simulink model "Copy_of_newCommunication"  (R2025a)
settings: Solver=VariableStepAuto  StartTime=0.0  StopTime=Inf  RelTol=1e-3
values from neighbouring files (symbols this model uses):
  Boom_Cmd_LUT = joints(1).lut_y    [LUT.m]
  Boom_Vel_LUT = joints(1).lut_x    [LUT.m]
  Stick_Cmd_LUT = joints(2).lut_y    [LUT.m]
  Stick_Vel_LUT = joints(2).lut_x    [LUT.m]
undefined symbols (not defined in the file or in its folder): canChannel
libraries: canlib x10, canmsglib x8, simulink x8, eeGeneralControl x5, simulink_extras x4, slpidlib x2, sl3dlib x1
settings Model: Creator=Viktor Traktor  LastModifiedBy=Viktor Traktor

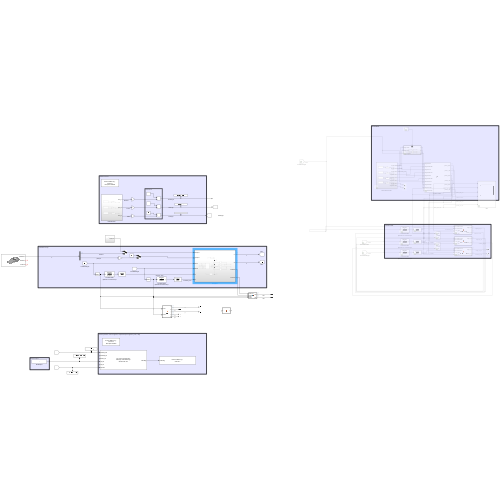
[thumbnail: Simulink's stored preview of the top-level diagram]
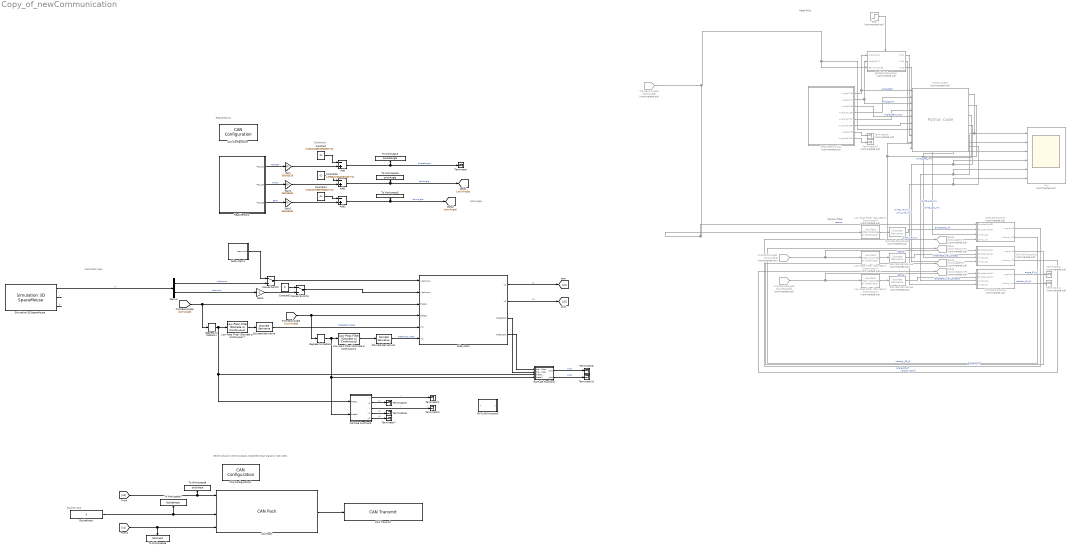
== system Copy_of_newCommunication ==
  note: Controller Loop
  note: bomAngle
  note: Calibration
  note: Send hydraulic control signals, expected input signals [-100, 100]
  note: Read sensors
  note: Bucket Input
  note: Kalman Filter
  note: Read IMUs
  Add : Sum  Inputs=-+
  Add1 : Sum  Inputs=-+
  Add2 : Sum  Inputs=-+
  BucketInput : Constant  Value=0
  CAN Configuration : canlib/CAN Configuration  BlockHandle=17154.0007  Device=Kvaser USBcan Light 1 (Channel 1)  DeviceMenu=Kvaser USBcan Light 1 (Channel 1)  ObjConstructor=canChannel('Kvaser', 'USBcan Light 1', 1)  BusSpeed=500000  EnableBitParameters=off  SJW=1  TSEG1=4  TSEG2=3  NSamples=1  AckMode=Normal
  CAN Configuration1 : canlib/CAN Configuration  BlockHandle=17155.0007  Device=Kvaser USBcan Light 1 (Channel 2)  DeviceMenu=Kvaser USBcan Light 1 (Channel 2)  ObjConstructor=canChannel('Kvaser', 'USBcan Light 1', 2)  BusSpeed=500000  EnableBitParameters=off  SJW=1  TSEG1=4  TSEG2=3  NSamples=1  AckMode=Normal
  CAN Pack : canmsglib/CAN Pack  CANdbFile=C:\Users\Viktor Traktor\IQAN\ec20_hydraulics.dbc  MsgList=ControlMessage  MsgName=ControlMessage  MsgIDType=Standard (11-bit identifier)  MsgIdentifier=387  CANIDInput=off  MsgLength=6  Remote=off  ApplyMinMax=off  BusOutput=off  SignalInfo={'Parallell_FR','8','8','LE','signed','Standard','0','1','0','-Inf','Inf';'Parallelll_RL','0','8','LE','signed','Standard','0','1','0','-Inf','Inf';'Rotate_RL','40','8','LE','signed','Standard','0','1','0','-Inf','Inf';'Tilt_FR','24','8','LE','signed','Standard','0','1','0','-Inf','Inf';'Tilt_RL','32','8','LE','signed','Standard','0','1','0','-Inf','Inf';'UpDown','16','8','LE','signed','Standard','0','1','0','-Inf','Inf'}
      settings: LibrarySourceBlock=canlib/CAN Pack  DataFormat=CANdb specified signals
  CAN Transmit : canlib/CAN Transmit  BlockHandle=17164.0007  Device=Kvaser USBcan Light 1 (Channel 2)  DeviceMenu=Kvaser USBcan Light 1 (Channel 2)  ObjConstructor=canChannel('Kvaser', 'USBcan Light 1', 2)  EnableEventTransmit=off  EnablePeriodicTransmit=off  MessagePeriod=1.000
  Constant : Constant  Value=2.060410383456638e+02
  Constant1 : Constant  Value=2.052407368979854e+02
  Constant2 : Constant  Value=0
  Constant5 : Constant  Value=2.390501084826040e+02
  Degrees to Radians : simulink_extras/Transformations/Degrees to Radians
  Degrees to Radians1 : simulink_extras/Transformations/Degrees to Radians
  Demux : Demux  Outputs=2
  Discrete Derivative : simulink/Discrete/Discrete Derivative  gainval=1.0  ICPrevScaledInput=0.0  OutMin=[]  OutMax=[]  OutDataType=fixdt(1, 16)  OutScaling=2^-10  DoSatur=off
  Discrete Derivative1 : simulink/Discrete/Discrete Derivative  gainval=1.0  ICPrevScaledInput=0.0  OutMin=[]  OutMax=[]  OutDataType=fixdt(1, 16)  OutScaling=2^-10  DoSatur=off
  Discrete Derivative2 : simulink/Discrete/Discrete Derivative  Commented=on  gainval=1.0  ICPrevScaledInput=0.0  OutMin=[]  OutMax=[]  OutDataType=fixdt(1, 16)  OutScaling=2^-10  DoSatur=off
  Discrete Derivative3 : simulink/Discrete/Discrete Derivative  Commented=on  gainval=1.0  ICPrevScaledInput=0.0  OutMin=[]  OutMax=[]  OutDataType=fixdt(1, 16)  OutScaling=2^-10  DoSatur=off
  Discrete Derivative4 : simulink/Discrete/Discrete Derivative  Commented=on  gainval=1.0  ICPrevScaledInput=0.0  OutMin=[]  OutMax=[]  OutDataType=fixdt(1, 16)  OutScaling=2^-10  DoSatur=off
  Enabled Subsystem : Subsystem  Commented=on  TreatAsAtomicUnit=on
  FromBomAngle1 : From  Commented=on  GotoTag=bomAngle
  FromBucketAngle : From  Commented=on  GotoTag=bucketAngle
  FromStickAngle1 : From  Commented=on  GotoTag=stickAngle
  Gain : Gain  Gain=360/65535
  Gain1 : Gain  Gain=360/65535
  Gain2 : Gain  Gain=360/65535
  Gain3 : Gain  Gain=-1
  Goto3 : Goto  Commented=on  GotoTag=bomAngleKF
  Goto4 : Goto  Commented=on  GotoTag=bomVelocityKF
  Goto5 : Goto  Commented=on  GotoTag=stickAngleKF
  Goto6 : Goto  Commented=on  GotoTag=stickVelocityKF
  IMU : Scope  Commented=on  NumInputPorts=6
      settings: ActiveDisplayYMinimum=240.03476604985391  ActiveDisplayYMaximum=241.62685406904103
  Low-Pass Filter (Discrete or Continuous)1 : eeGeneralControl/Low-Pass Filter (Discrete or Continuous)  K=1  T=.15  B=inf  A=-inf  init_option=Inherited from block input  x0=0  Ts=0.1
  Low-Pass Filter (Discrete or Continuous)4 : eeGeneralControl/Low-Pass Filter (Discrete or Continuous)  Commented=on  K=1  T=.15  B=inf  A=-inf  init_option=Inherited from block input  x0=0  Ts=0.1
  Low-Pass Filter (Discrete or Continuous)5 : eeGeneralControl/Low-Pass Filter (Discrete or Continuous)  Commented=on  K=1  T=.15  B=inf  A=-inf  init_option=Inherited from block input  x0=0  Ts=0.1
  Low-Pass Filter (Discrete or Continuous)6 : eeGeneralControl/Low-Pass Filter (Discrete or Continuous)  Commented=on  K=1  T=.15  B=inf  A=-inf  init_option=Inherited from block input  x0=0  Ts=0.1
  Low-Pass Filter (Discrete or Continuous)7 : eeGeneralControl/Low-Pass Filter (Discrete or Continuous)  K=1  T=.15  B=inf  A=-inf  init_option=Inherited from block input  x0=0  Ts=0.1
  MATLAB Function : MATLAB Function  Commented=on  TreatAsAtomicUnit=on
  MATLAB Function1 : MATLAB Function  Commented=on  TreatAsAtomicUnit=on
  MATLAB Function2 : MATLAB Function  Commented=on  TreatAsAtomicUnit=on
  MATLAB Function3 : MATLAB Function  TreatAsAtomicUnit=on
  MATLAB Function4 : MATLAB Function  TreatAsAtomicUnit=on
  MATLAB Function5 : MATLAB Function  TreatAsAtomicUnit=on
  Manual Switch : ManualSwitch
  Manual Switch1 : ManualSwitch
  Python Code1 : PythonCode  Commented=on  OutputCode=|  SampleTime=0.01
      | # Computation
      | 
      | #print(Angle128X)
      | 
      | if Angle128X > 180:
      |     Angle128X = abs(Angle128X) - 360
      |     
      | if Angle137X < 20:
      |     Angle137X = abs(Angle137X)+360
      |     
      | if Angle138X > 270:
      |     Angle138X = abs(Angle138X) - 360
      |     
      | #print("///")
      | #print(Angle128X)
      | 
      | print(Angle128Xp)
      | print(Angle137Xp)
      | print(Encoder33Xp)
      |     
      | joint1_pos = Angle137X -270 + Angle128X - (Angle137Xp-270 + Angle128Xp - Encoder33Xp)
      | joint1_vel = -(AngleVel137X - AngleVel128X)
      | 
      | joint2_pos = 180 + (90 - joint1_pos) + Angle138X
      | joint2_vel = AngleVel138X - joint1_vel
      | 
      | joint3_pos = 0
      | joint3_vel = 0
  Read Sensors : Subsystem
  Read Sensors IMU : Subsystem  Commented=on
  Simulation 3D SpaceMouse : sl3dlib/Simulation 3D/Hardware Interface/Simulation 3D SpaceMouse  Port=USB1  OutputType=Speed  Dominant=off  DisableTranslation=off  DisableRotation=off  NormalizeAngle=off  EnableLimit=off  PositionSensitivity=0.00058  RotationSensitivity=0.00001  InitialPosition=[0 0 0]  InitialRotation=[0 0 1 0]  PositionLow=[-100 -100 -100]  PositionUp=[100 100 100]
  Step : Step  Commented=on  Time=0.001  Before=1  After=0  SampleTime=0
  Subsystem : Subsystem
  Subsystem1 : Subsystem
  Terminator{,1,3,5..8,11} (8 alike) : Terminator
  Terminator{2,4,9..10} (4 alike) : Terminator  Commented=on
  To Workspace : ToWorkspace  VariableName=bucketAngle  SaveFormat=Timeseries  SampleTime=-1
  To Workspace1 : ToWorkspace  VariableName=stickAngle  SaveFormat=Timeseries  SampleTime=-1
  To Workspace2 : ToWorkspace  VariableName=bomAngle  SaveFormat=Timeseries  SampleTime=-1
  To Workspace6 : ToWorkspace  VariableName=bomInput  SaveFormat=Timeseries  SampleTime=-1
  To Workspace7 : ToWorkspace  VariableName=bucketInput  SaveFormat=Timeseries  SampleTime=-1
  To Workspace8 : ToWorkspace  VariableName=stickInput  SaveFormat=Timeseries  SampleTime=-1
  wires:
  BucketInput/1 -> CAN Pack/4, To Workspace7/1
  Add2/1 -> [bomAngle], To Workspace2/1  "bomAngle"
  Constant1/1 -> Add2/1
  Gain/1 -> Add/2
  Read Sensors/2(Pos_20) -> Gain1/1  "STICK"
  [u2] -> CAN Pack/1, To Workspace8/1
  Constant/1 -> Add/1
  Read Sensors/1(Pos_01) -> Gain/1  "BUCKET"
  Gain2/1 -> Add2/2
  Read Sensors/3(Pos_33) -> Gain2/1  "BOM"
  CAN Pack/1 -> CAN Transmit/1
  Add/1 -> Terminator/1, To Workspace/1  "bucketAngle"
  [u1] -> CAN Pack/6, To Workspace6/1
  Add1/1 -> [stickAngle], To Workspace1/1  "stickAngle"
  MATLAB Function1/2(velocity_20) -> Goto6/1  "velocity_20_kf"
  Enabled Subsystem/1(Out1) -> Python Code1/8
  Discrete Derivative2/1 -> MATLAB Function/2(EncoderVel33X)  "Encoder33_vel"
  MATLAB Function/1(angle_33) -> Goto3/1  "angle_33_kf"
  Read Sensors IMU/3(Angle138X) -> Python Code1/5  "Angle138X_input"
  Python Code1/4 -> MATLAB Function1/4(joint2_vel), IMU/4  "join2_vel_imu"
  Read Sensors IMU/4(AngleVel128X) -> Python Code1/2
  Read Sensors IMU/1(Angle128X) -> Python Code1/1, Enabled Subsystem/1(Angle128X)  "Angle128X"
  Read Sensors IMU/8(AngleVel139X) -> Terminator10/1
  Python Code1/3 -> IMU/3, MATLAB Function1/3(joint2_pos)  "joint2_pos_imu"
  Python Code1/5 -> MATLAB Function2/3(joint3_pos), IMU/5  "joint3_pos_imu"
  MATLAB Function/2(velocity_33) -> Goto4/1  "velocity_33_kf"
  Python Code1/6 -> MATLAB Function2/4(joint3_vel), IMU/6  "joint3_vel_imu"
  Python Code1/2 -> IMU/2, MATLAB Function/4(joint1_vel)  "joint1_vel_imu"
  MATLAB Function1/1(angle_20) -> Goto5/1  "anlge_20_kf"
  Enabled Subsystem/3(Out3) -> Python Code1/10
  Read Sensors IMU/2(Angle137X) -> Python Code1/3, Enabled Subsystem/2(Angle137X)  "Angle137X"
  Step/1 -> Enabled Subsystem/Enable
  Discrete Derivative3/1 -> MATLAB Function1/2(EncoderVel20X)  "Encoder20_vel_Lowpass"
  Read Sensors IMU/5(AngleVel137X) -> Python Code1/4
  Python Code1/1 -> MATLAB Function/3(joint1_pos), IMU/1  "joint1_pos_imu"
  MATLAB Function2/1(angle_01) -> Terminator2/1  "angle_01_kf"
  Read Sensors IMU/7(Angle139X) -> Terminator9/1
  MATLAB Function2/2(velocity_01) -> Terminator4/1  "velocity_01_kf"
  Read Sensors IMU/6(AngleVel138X) -> Python Code1/6
  Enabled Subsystem/2(Out2) -> Python Code1/9
  Discrete Derivative4/1 -> MATLAB Function2/2(EncoderVel01X)  "Encoder01_vel_Lowpass"
  Constant5/1 -> Add1/1
  FromStickAngle1/1 -> MATLAB Function1/1(EncoderPos20X), Low-Pass Filter (Discrete or Continuous)4/1  "testvel"
  FromBomAngle1/1 -> Python Code1/7, Enabled Subsystem/3(BoomAngle33), Low-Pass Filter (Discrete or Continuous)6/1, MATLAB Function/1(EncoderPos33X)  "testvel"
  FromBucketAngle/1 -> MATLAB Function2/1(EncoderPos01X), Low-Pass Filter (Discrete or Continuous)5/1  "testvel"
  Low-Pass Filter (Discrete or Continuous)5/1 -> Discrete Derivative4/1
  Low-Pass Filter (Discrete or Continuous)4/1 -> Discrete Derivative3/1
  Low-Pass Filter (Discrete or Continuous)6/1 -> Discrete Derivative2/1
  Simulation 3D SpaceMouse/1 -> Demux/1  "tr"
  [stickAngle] -> Degrees to Radians/1, Subsystem/4(theta2)
  Low-Pass Filter (Discrete or Continuous)7/1 -> Discrete Derivative/1
  Discrete Derivative/1 -> Subsystem/5(In1)  "thetadot1_meas"
  Subsystem/2(u2) -> [u2]  "u2"
  [bomAngle] -> Degrees to Radians1/1, Subsystem/3(theta1)
  Low-Pass Filter (Discrete or Continuous)1/1 -> Discrete Derivative1/1
  Demux/2 -> Gain3/1  "ydotInput"
  Demux/1 -> Manual Switch/2  "xdotInput"
  Simulation 3D SpaceMouse/2 -> ?  "r"
  Simulation 3D SpaceMouse/3 -> ?  "b"
  Discrete Derivative1/1 -> Subsystem/6(In2)  "thetadot2_meas"
  Subsystem/1(u1) -> [u1]  "u1"
  Degrees to Radians/1 -> MATLAB Function3/2(theta2), MATLAB Function4/4(theta2), Low-Pass Filter (Discrete or Continuous)1/1
  Gain3/1 -> Manual Switch1/2
  MATLAB Function3/1(x) -> Terminator1/1  "x"
  MATLAB Function3/3(y) -> Terminator3/1  "y"
  Degrees to Radians1/1 -> MATLAB Function4/3(theta1), MATLAB Function3/1(theta1), Low-Pass Filter (Discrete or Continuous)7/1
  MATLAB Function3/2(x1) -> Terminator5/1  "x1"
  MATLAB Function3/4(y1) -> Terminator6/1  "y1"
  MATLAB Function3/5(y2) -> Terminator7/1  "y2"
  Gain1/1 -> Add1/2
  Subsystem1/1(stepInput) -> Manual Switch/1
  Constant2/1 -> Manual Switch1/1
  Manual Switch/1 -> Subsystem/1(xdotInput)
  Manual Switch1/1 -> Subsystem/2(ydotInput)
  MATLAB Function4/1(xdot) -> Terminator8/1  "xdot"
  MATLAB Function4/2(ydot) -> Terminator11/1  "ydot"
  Subsystem/4(theta1dot) -> MATLAB Function4/1(theta1dot)
  Subsystem/3(theta2dot) -> MATLAB Function4/2(theta2dot)

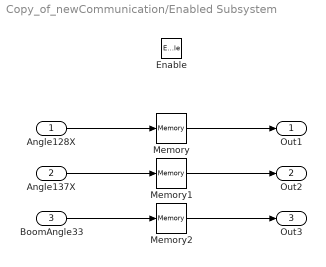
== system Copy_of_newCommunication/Enabled Subsystem ==
  Angle128X : Inport
  Angle137X : Inport  Port=2
  BoomAngle33 : Inport  Port=3
  Enable : EnablePort
  Memory : Memory
  Memory1 : Memory
  Memory2 : Memory
  Out1 : Outport
  Out2 : Outport  Port=2
  Out3 : Outport  Port=3
  wires:
  Angle128X/1 -> Memory/1
  Memory/1 -> Out1/1
  Angle137X/1 -> Memory1/1
  BoomAngle33/1 -> Memory2/1
  Memory1/1 -> Out2/1
  Memory2/1 -> Out3/1

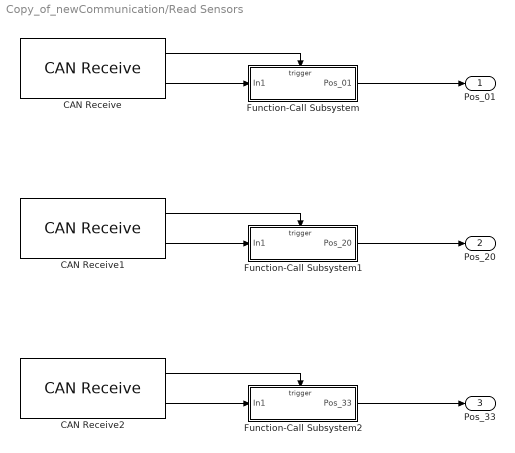
== system Copy_of_newCommunication/Read Sensors ==
  CAN Receive : canlib/CAN Receive  BlockHandle=17549.0105  Device=Kvaser USBcan Light 1 (Channel 1)  DeviceMenu=Kvaser USBcan Light 1 (Channel 1)  ObjConstructor=canChannel('Kvaser', 'USBcan Light 1', 1)  EnableStandardIDsFilter=off  StdIDsCombo=Allow all  StandardIDs=0  EnableExtendedIDsFilter=off  ExtIDsCombo=Allow all  ExtendedIDs=0  SampleTime=0.01  MsgsPerTimestep=all  InternalFilterUpdateStatus=on  BusOutput=off
  CAN Receive1 : canlib/CAN Receive  BlockHandle=17552.0105  Device=Kvaser USBcan Light 1 (Channel 1)  DeviceMenu=Kvaser USBcan Light 1 (Channel 1)  ObjConstructor=canChannel('Kvaser', 'USBcan Light 1', 1)  EnableStandardIDsFilter=off  StdIDsCombo=Allow all  StandardIDs=0  EnableExtendedIDsFilter=off  ExtIDsCombo=Allow all  ExtendedIDs=0  SampleTime=0.01  MsgsPerTimestep=all  InternalFilterUpdateStatus=on  BusOutput=off
  CAN Receive2 : canlib/CAN Receive  BlockHandle=17555.0105  Device=Kvaser USBcan Light 1 (Channel 1)  DeviceMenu=Kvaser USBcan Light 1 (Channel 1)  ObjConstructor=canChannel('Kvaser', 'USBcan Light 1', 1)  EnableStandardIDsFilter=off  StdIDsCombo=Allow all  StandardIDs=0  EnableExtendedIDsFilter=off  ExtIDsCombo=Allow all  ExtendedIDs=0  SampleTime=0.01  MsgsPerTimestep=all  InternalFilterUpdateStatus=on  BusOutput=off
  Function-Call Subsystem : Subsystem  TreatAsAtomicUnit=on
  Function-Call Subsystem1 : Subsystem  TreatAsAtomicUnit=on
  Function-Call Subsystem2 : Subsystem  TreatAsAtomicUnit=on
  Pos_01 : Outport
  Pos_20 : Outport  Port=2
  Pos_33 : Outport  Port=3
  wires:
  CAN Receive/2 -> Function-Call Subsystem/1(In1)
  CAN Receive1/2 -> Function-Call Subsystem1/1(In1)
  CAN Receive/1 -> Function-Call Subsystem/Trigger
  CAN Receive2/2 -> Function-Call Subsystem2/1(In1)
  Function-Call Subsystem2/1(Pos_33) -> Pos_33/1
  Function-Call Subsystem/1(Pos_01) -> Pos_01/1
  CAN Receive2/1 -> Function-Call Subsystem2/Trigger
  CAN Receive1/1 -> Function-Call Subsystem1/Trigger
  Function-Call Subsystem1/1(Pos_20) -> Pos_20/1

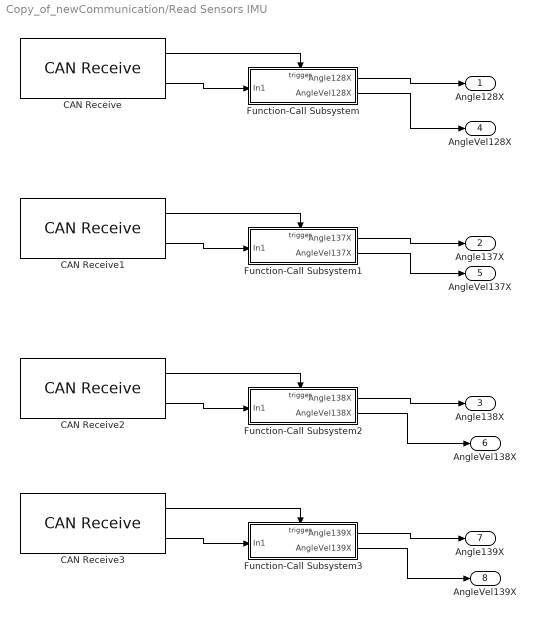
== system Copy_of_newCommunication/Read Sensors IMU ==
  CAN Receive : canlib/CAN Receive  BlockHandle=776.0005  Device=MathWorks Virtual 1 (Channel 1)  DeviceMenu=MathWorks Virtual 1 (Channel 1)  ObjConstructor=canChannel('MathWorks', 'Virtual 1', 1)  EnableStandardIDsFilter=off  StdIDsCombo=Allow all  StandardIDs=0  EnableExtendedIDsFilter=off  ExtIDsCombo=Allow all  ExtendedIDs=0  SampleTime=0.01  MsgsPerTimestep=all  InternalFilterUpdateStatus=on  BusOutput=off
  CAN Receive1 : canlib/CAN Receive  BlockHandle=779.0005  Device=MathWorks Virtual 1 (Channel 1)  DeviceMenu=MathWorks Virtual 1 (Channel 1)  ObjConstructor=canChannel('MathWorks', 'Virtual 1', 1)  EnableStandardIDsFilter=off  StdIDsCombo=Allow all  StandardIDs=0  EnableExtendedIDsFilter=off  ExtIDsCombo=Allow all  ExtendedIDs=0  SampleTime=0.01  MsgsPerTimestep=all  InternalFilterUpdateStatus=on  BusOutput=off
  CAN Receive2 : canlib/CAN Receive  BlockHandle=782.0005  Device=MathWorks Virtual 1 (Channel 1)  DeviceMenu=MathWorks Virtual 1 (Channel 1)  ObjConstructor=canChannel('MathWorks', 'Virtual 1', 1)  EnableStandardIDsFilter=off  StdIDsCombo=Allow all  StandardIDs=0  EnableExtendedIDsFilter=off  ExtIDsCombo=Allow all  ExtendedIDs=0  SampleTime=0.01  MsgsPerTimestep=all  InternalFilterUpdateStatus=on  BusOutput=off
  CAN Receive3 : canlib/CAN Receive  BlockHandle=785.0005  Device=MathWorks Virtual 1 (Channel 1)  DeviceMenu=MathWorks Virtual 1 (Channel 1)  ObjConstructor=canChannel('MathWorks', 'Virtual 1', 1)  EnableStandardIDsFilter=off  StdIDsCombo=Allow all  StandardIDs=0  EnableExtendedIDsFilter=off  ExtIDsCombo=Allow all  ExtendedIDs=0  SampleTime=0.01  MsgsPerTimestep=all  InternalFilterUpdateStatus=on  BusOutput=off
  Function-Call Subsystem : Subsystem  TreatAsAtomicUnit=on
  Function-Call Subsystem1 : Subsystem  TreatAsAtomicUnit=on
  Function-Call Subsystem2 : Subsystem  TreatAsAtomicUnit=on
  Function-Call Subsystem3 : Subsystem  TreatAsAtomicUnit=on
  Angle128X : Outport
  Angle137X : Outport  Port=2
  Angle138X : Outport  Port=3
  AngleVel128X : Outport  Port=4
  AngleVel137X : Outport  Port=5
  AngleVel138X : Outport  Port=6
  Angle139X : Outport  Port=7
  AngleVel139X : Outport  Port=8
  wires:
  Function-Call Subsystem1/1(Angle137X) -> Angle137X/1
  CAN Receive1/1 -> Function-Call Subsystem1/Trigger
  CAN Receive2/1 -> Function-Call Subsystem2/Trigger
  Function-Call Subsystem/1(Angle128X) -> Angle128X/1
  Function-Call Subsystem2/1(Angle138X) -> Angle138X/1
  CAN Receive2/2 -> Function-Call Subsystem2/1(In1)
  CAN Receive/1 -> Function-Call Subsystem/Trigger
  CAN Receive1/2 -> Function-Call Subsystem1/1(In1)
  CAN Receive/2 -> Function-Call Subsystem/1(In1)
  Function-Call Subsystem/2(AngleVel128X) -> AngleVel128X/1
  Function-Call Subsystem1/2(AngleVel137X) -> AngleVel137X/1
  Function-Call Subsystem2/2(AngleVel138X) -> AngleVel138X/1
  Function-Call Subsystem3/2(AngleVel139X) -> AngleVel139X/1
  CAN Receive3/2 -> Function-Call Subsystem3/1(In1)
  Function-Call Subsystem3/1(Angle139X) -> Angle139X/1
  CAN Receive3/1 -> Function-Call Subsystem3/Trigger

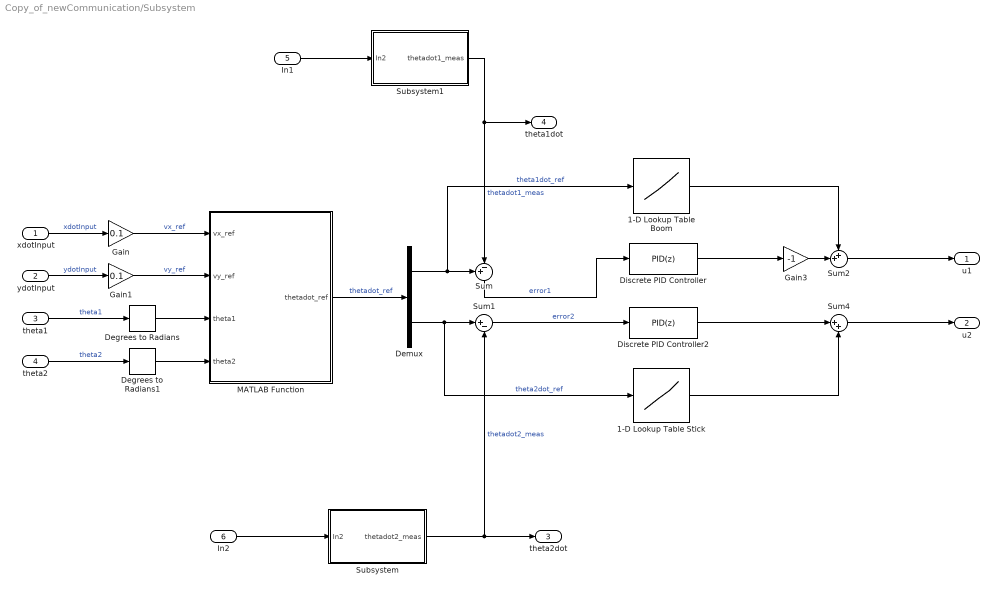
== system Copy_of_newCommunication/Subsystem ==
  xdotInput : Inport
  ydotInput : Inport  Port=2
  theta1 : Inport  Port=3
  theta2 : Inport  Port=4
  In1 : Inport  Port=5
  In2 : Inport  Port=6
  1-D Lookup Table Boom : Lookup_n-D  NumberOfTableDimensions=1  BreakpointsForDimension1=Boom_Vel_LUT  Table=Boom_Cmd_LUT  InternalRulePriority=Speed  RndMeth=Simplest
  1-D Lookup Table Stick : Lookup_n-D  NumberOfTableDimensions=1  BreakpointsForDimension1=Stick_Vel_LUT  Table=Stick_Cmd_LUT  InternalRulePriority=Speed  RndMeth=Simplest
  Degrees to Radians : simulink_extras/Transformations/Degrees to Radians
  Degrees to Radians1 : simulink_extras/Transformations/Degrees to Radians
  Demux : Demux  Outputs=2
  Discrete PID Controller : slpidlib/PID Controller  Controller=PID  Form=Parallel  TimeDomain=Discrete-time  UseExternalTs=off  SampleTime=-1  IntegratorMethod=Forward Euler  FilterMethod=Forward Euler  ControllerParametersSource=internal  P=1  I=0  UseKiTs=off  D=0  UseExternalDerivativeSource=off  N=100  UseFilter=on  TunerSelectOption=Transfer Function Based (PID Tuner App)  InitialConditionSource=internal  InitialConditionForIntegrator=0  InitialConditionForFilter=0  DifferentiatorICPrevScaledInput=0  ExternalReset=none  TrackingMode=off  Kt=1  LimitOutput=on  SatLimitsSource=internal  UpperSaturationLimit=100  LowerSaturationLimit=-100  LinearizeAsGain=off  AntiWindupMode=clamping  Kb=1  LimitIntegrator=on  UpperIntegratorSaturationLimit=50  LowerIntegratorSaturationLimit=-50  POutMin=[]  POutMax=[]  IOutMin=[]  IOutMax=[]  DOutMin=[]  DOutMax=[]  NOutMin=[]  NOutMax=[]  SumOutMin=[]  SumOutMax=[]  SaturationOutMin=[]  SaturationOutMax=[]  PParamMin=[]  PParamMax=[]  IParamMin=[]  IParamMax=[]  DParamMin=[]  DParamMax=[]  NParamMin=[]  NParamMax=[]  KbParamMin=[]  KbParamMax=[]  KtParamMin=[]  KtParamMax=[]  KbOutMin=[]  KbOutMax=[]  KtOutMin=[]  KtOutMax=[]  IntegratorOutMin=[]  IntegratorOutMax=[]  FilterOutMin=[]  FilterOutMax=[]  SumI1OutMin=[]  SumI1OutMax=[]  SumI2OutMin=[]  SumI2OutMax=[]  SumI3OutMin=[]  SumI3OutMax=[]  SumI4OutMin=[]  SumI4OutMax=[]  SumDOutMin=[]  SumDOutMax=[]  DifferentiatorOutMin=[]  DifferentiatorOutMax=[]  FilterDiffOutCoefMin=[]  FilterDiffOutCoefMax=[]  ReciprocalOutMin=[]  ReciprocalOutMax=[]  SumDenOutMin=[]  SumDenOutMax=[]  SumNumOutMin=[]  SumNumOutMax=[]  DivideOutMin=[]  DivideOutMax=[]  UdiffTsProdOutMin=[]  UdiffTsProdOutMax=[]  NTsProdOutMin=[]  NTsProdOutMax=[]  UintegralTsProdOutMin=[]  UintegralTsProdOutMax=[]  UngainTsProdOutMin=[]  UngainTsProdOutMax=[]  ClampingZeroOutDataTypeStr=Inherit: Inherit via back propagation  ClampingZeroOutMin=[]  ClampingZeroOutMax=[]  FilterDenConstantOutDataTypeStr=Inherit: Inherit via back propagation  FilterDenConstantOutMin=[]  FilterDenConstantOutMax=[]  PCopyOutDataTypeStr=Inherit: Inherit via back propagation  PCopyOutMin=[]  PCopyOutMax=[]  NCopyOutDataTypeStr=Inherit: Inherit via back propagation  NCopyOutMin=[]  NCopyOutMax=[]  IntegratorContinuousStateAttributes=''  IntegratorStateMustResolveToSignalObject=off  IntegratorRTWStateStorageClass=Auto  FilterContinuousStateAttributes=''  FilterStateMustResolveToSignalObject=off  FilterRTWStateStorageClass=Auto  ParallelPVariant=InternalParameters  IdealPVariant=Disabled  IVariant=InternalParameters  DVariant=InternalParameters  IntegratorVariant=Discrete  SatVariant=Enabled  AWVariant=DiscClampingParallel  PCopyVariant=Disabled  TRVariant=Disabled  FdbkBlocksVariant=Forward  IdealPFdbkVariant=Disabled  SatFdbkVariant=Disabled  DerivativeFilterVariant=ForwardEulerFilter  NVariant=InternalParameters  NCopyVariant=Disabled  FilterICVariant=InternalICsFilter  IntegratorICVariant=InternalICs  ExternalResetVariant=Disabled  TRSumVariant=Passthrough  SumFdbkVariant=Disabled  SumVariant=Sum_PID  TsampFilterVariant=InternalTs  TsampNgainVariant=Passthrough  TsampIntegralVariant=Disabled_SignalSpec  ExternalSaturationOutDataTypeStr=Inherit: Same as second input  DerivativeSourceVariant=ErrorSignal  PreIntVariant=InternalPreInt
      settings: LibrarySourceBlock=simulink/Discrete/Discrete PID Controller
  Discrete PID Controller2 : slpidlib/PID Controller  Controller=PID  Form=Parallel  TimeDomain=Discrete-time  UseExternalTs=off  SampleTime=-1  IntegratorMethod=Forward Euler  FilterMethod=Forward Euler  ControllerParametersSource=internal  P=1  I=0  UseKiTs=off  D=0  UseExternalDerivativeSource=off  N=100  UseFilter=on  TunerSelectOption=Transfer Function Based (PID Tuner App)  InitialConditionSource=internal  InitialConditionForIntegrator=0  InitialConditionForFilter=0  DifferentiatorICPrevScaledInput=0  ExternalReset=none  TrackingMode=off  Kt=1  LimitOutput=on  SatLimitsSource=internal  UpperSaturationLimit=100  LowerSaturationLimit=-100  LinearizeAsGain=off  AntiWindupMode=clamping  Kb=1  LimitIntegrator=on  UpperIntegratorSaturationLimit=50  LowerIntegratorSaturationLimit=-50  POutMin=[]  POutMax=[]  IOutMin=[]  IOutMax=[]  DOutMin=[]  DOutMax=[]  NOutMin=[]  NOutMax=[]  SumOutMin=[]  SumOutMax=[]  SaturationOutMin=[]  SaturationOutMax=[]  PParamMin=[]  PParamMax=[]  IParamMin=[]  IParamMax=[]  DParamMin=[]  DParamMax=[]  NParamMin=[]  NParamMax=[]  KbParamMin=[]  KbParamMax=[]  KtParamMin=[]  KtParamMax=[]  KbOutMin=[]  KbOutMax=[]  KtOutMin=[]  KtOutMax=[]  IntegratorOutMin=[]  IntegratorOutMax=[]  FilterOutMin=[]  FilterOutMax=[]  SumI1OutMin=[]  SumI1OutMax=[]  SumI2OutMin=[]  SumI2OutMax=[]  SumI3OutMin=[]  SumI3OutMax=[]  SumI4OutMin=[]  SumI4OutMax=[]  SumDOutMin=[]  SumDOutMax=[]  DifferentiatorOutMin=[]  DifferentiatorOutMax=[]  FilterDiffOutCoefMin=[]  FilterDiffOutCoefMax=[]  ReciprocalOutMin=[]  ReciprocalOutMax=[]  SumDenOutMin=[]  SumDenOutMax=[]  SumNumOutMin=[]  SumNumOutMax=[]  DivideOutMin=[]  DivideOutMax=[]  UdiffTsProdOutMin=[]  UdiffTsProdOutMax=[]  NTsProdOutMin=[]  NTsProdOutMax=[]  UintegralTsProdOutMin=[]  UintegralTsProdOutMax=[]  UngainTsProdOutMin=[]  UngainTsProdOutMax=[]  ClampingZeroOutDataTypeStr=Inherit: Inherit via back propagation  ClampingZeroOutMin=[]  ClampingZeroOutMax=[]  FilterDenConstantOutDataTypeStr=Inherit: Inherit via back propagation  FilterDenConstantOutMin=[]  FilterDenConstantOutMax=[]  PCopyOutDataTypeStr=Inherit: Inherit via back propagation  PCopyOutMin=[]  PCopyOutMax=[]  NCopyOutDataTypeStr=Inherit: Inherit via back propagation  NCopyOutMin=[]  NCopyOutMax=[]  IntegratorContinuousStateAttributes=''  IntegratorStateMustResolveToSignalObject=off  IntegratorRTWStateStorageClass=Auto  FilterContinuousStateAttributes=''  FilterStateMustResolveToSignalObject=off  FilterRTWStateStorageClass=Auto  ParallelPVariant=InternalParameters  IdealPVariant=Disabled  IVariant=InternalParameters  DVariant=InternalParameters  IntegratorVariant=Discrete  SatVariant=Enabled  AWVariant=DiscClampingParallel  PCopyVariant=Disabled  TRVariant=Disabled  FdbkBlocksVariant=Forward  IdealPFdbkVariant=Disabled  SatFdbkVariant=Disabled  DerivativeFilterVariant=ForwardEulerFilter  NVariant=InternalParameters  NCopyVariant=Disabled  FilterICVariant=InternalICsFilter  IntegratorICVariant=InternalICs  ExternalResetVariant=Disabled  TRSumVariant=Passthrough  SumFdbkVariant=Disabled  SumVariant=Sum_PID  TsampFilterVariant=InternalTs  TsampNgainVariant=Passthrough  TsampIntegralVariant=Disabled_SignalSpec  ExternalSaturationOutDataTypeStr=Inherit: Same as second input  DerivativeSourceVariant=ErrorSignal  PreIntVariant=InternalPreInt
      settings: LibrarySourceBlock=simulink/Discrete/Discrete PID Controller
  Gain : Gain  Gain=0.1
  Gain1 : Gain  Gain=0.1
  Gain3 : Gain  Gain=-1
  MATLAB Function : MATLAB Function  TreatAsAtomicUnit=on
  Subsystem : Subsystem
  Subsystem1 : Subsystem
  Sum : Sum  Inputs=+-|
  Sum1 : Sum  Inputs=|+-
  Sum2 : Sum  Inputs=++|
  Sum4 : Sum  Inputs=|++
  u1 : Outport
  u2 : Outport  Port=2
  theta2dot : Outport  Port=3
  theta1dot : Outport  Port=4
  wires:
  Sum/1 -> Discrete PID Controller/1  "error1"
  MATLAB Function/1(thetadot_ref) -> Demux/1  "thetadot_ref"
  xdotInput/1 -> Gain/1  "xdotInput"
  ydotInput/1 -> Gain1/1  "ydotInput"
  theta1/1 -> Degrees to Radians/1  "theta1"
  theta2/1 -> Degrees to Radians1/1  "theta2"
  Demux/1 -> 1-D Lookup Table Boom/1, Sum/1  "theta1dot_ref"
  In1/1 -> Subsystem1/1(In2)
  Demux/2 -> 1-D Lookup Table Stick/1, Sum1/1  "theta2dot_ref"
  Sum1/1 -> Discrete PID Controller2/1  "error2"
  Gain/1 -> MATLAB Function/1(vx_ref)  "vx_ref"
  Gain1/1 -> MATLAB Function/2(vy_ref)  "vy_ref"
  In2/1 -> Subsystem/1(In2)
  Subsystem/1(thetadot2_meas) -> theta2dot/1, Sum1/2  "thetadot2_meas"
  Subsystem1/1(thetadot1_meas) -> theta1dot/1, Sum/2  "thetadot1_meas"
  Degrees to Radians/1 -> MATLAB Function/3(theta1)
  Degrees to Radians1/1 -> MATLAB Function/4(theta2)
  Discrete PID Controller2/1 -> Sum4/1
  Gain3/1 -> Sum2/2
  Discrete PID Controller/1 -> Gain3/1
  Sum4/1 -> u2/1
  Sum2/1 -> u1/1
  1-D Lookup Table Boom/1 -> Sum2/1
  1-D Lookup Table Stick/1 -> Sum4/2

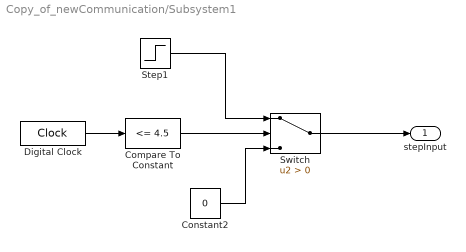
== system Copy_of_newCommunication/Subsystem1 ==
  Compare To Constant : simulink/Logic and Bit Operations/Compare To Constant  relop=<=  const=4.5  OutDataTypeStr=boolean
  Constant2 : Constant  Value=0
  Digital Clock : DigitalClock  SampleTime=0.01
  Step1 : Step  After=-1  SampleTime=0.01
  Switch : Switch  Criteria=u2 > Threshold  SaturateOnIntegerOverflow=off  InputSameDT=off
  stepInput : Outport
  wires:
  Switch/1 -> stepInput/1
  Compare To Constant/1 -> Switch/2
  Digital Clock/1 -> Compare To Constant/1
  Step1/1 -> Switch/1
  Constant2/1 -> Switch/3

== system Copy_of_newCommunication/Read Sensors/Function-Call Subsystem ==
  In1 : Inport
  function : TriggerPort  TriggerType=function-call  VariantControl=(inherit)
  CAN Unpack : canmsglib/CAN Unpack  CANdbFile=C:\Users\Viktor Traktor\Downloads\VolvoExcavator\systemIdentificationVolvo\ec20_kth.dbc  MsgList=Rot_01  MsgName=Rot_01  MsgIDType=Extended (29-bit identifier)  MsgIdentifier=419408385  MsgLength=8  SignalInfo={'SnsrPos_01','0','32','LE','unsigned','Standard','0','1','0','0','4294967295';'SnsrRPM_01','32','16','LE','unsigned','Standard','0','1','0','0','65535'}  IDPort=off  TimestampPort=off  ErrorPort=off  RemotePort=off  LengthPort=off  StatusPort=off  ApplyMinMax=off
      settings: LibrarySourceBlock=canlib/CAN Unpack  DataFormat=CANdb specified signals
  Terminator : Terminator
  Pos_01 : Outport
  wires:
  In1/1 -> CAN Unpack/1
  CAN Unpack/1 -> Pos_01/1
  CAN Unpack/2 -> Terminator/1

== system Copy_of_newCommunication/Read Sensors/Function-Call Subsystem1 ==
  In1 : Inport
  function : TriggerPort  TriggerType=function-call  VariantControl=(inherit)
  CAN Unpack : canmsglib/CAN Unpack  CANdbFile=C:\Users\Viktor Traktor\Downloads\VolvoExcavator\systemIdentificationVolvo\ec20_kth.dbc  MsgList=Rot_20  MsgName=Rot_20  MsgIDType=Extended (29-bit identifier)  MsgIdentifier=419408416  MsgLength=8  SignalInfo={'SnsrPos_20','0','32','LE','unsigned','Standard','0','1','0','0','4294967295';'SnsrRPM_20','32','16','LE','unsigned','Standard','0','1','0','0','65535'}  IDPort=off  TimestampPort=off  ErrorPort=off  RemotePort=off  LengthPort=off  StatusPort=off  ApplyMinMax=off
      settings: LibrarySourceBlock=canlib/CAN Unpack  DataFormat=CANdb specified signals
  Terminator : Terminator
  Pos_20 : Outport
  wires:
  CAN Unpack/1 -> Pos_20/1
  In1/1 -> CAN Unpack/1
  CAN Unpack/2 -> Terminator/1

== system Copy_of_newCommunication/Read Sensors/Function-Call Subsystem2 ==
  In1 : Inport
  function : TriggerPort  TriggerType=function-call  VariantControl=(inherit)
  CAN Unpack : canmsglib/CAN Unpack  CANdbFile=C:\Users\Viktor Traktor\Downloads\VolvoExcavator\systemIdentificationVolvo\ec20_kth.dbc  MsgList=Rot_33  MsgName=Rot_33  MsgIDType=Extended (29-bit identifier)  MsgIdentifier=419408435  MsgLength=8  SignalInfo={'SnsrPos_33','0','32','LE','unsigned','Standard','0','1','0','0','4294967295';'SnsrRPM_33','32','16','LE','unsigned','Standard','0','1','0','0','65535'}  IDPort=off  TimestampPort=off  ErrorPort=off  RemotePort=off  LengthPort=off  StatusPort=off  ApplyMinMax=off
      settings: LibrarySourceBlock=canlib/CAN Unpack  DataFormat=CANdb specified signals
  Terminator : Terminator
  Pos_33 : Outport
  wires:
  In1/1 -> CAN Unpack/1
  CAN Unpack/1 -> Pos_33/1
  CAN Unpack/2 -> Terminator/1

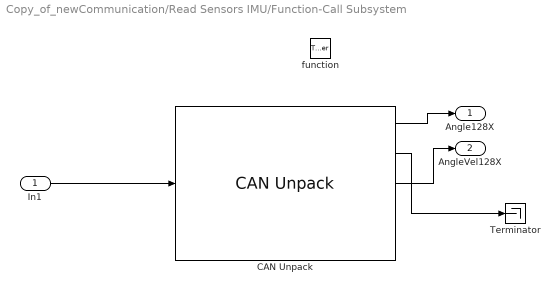
== system Copy_of_newCommunication/Read Sensors IMU/Function-Call Subsystem ==
  In1 : Inport
  function : TriggerPort  TriggerType=function-call  VariantControl=(inherit)
  CAN Unpack : canmsglib/CAN Unpack  CANdbFile=C:\Users\Viktor Traktor\Downloads\VolvoExcavator\systemIdentificationVolvo\ec20_kth.dbc  MsgList=IMU_XAxis_128  MsgName=IMU_XAxis_128  MsgIDType=Extended (29-bit identifier)  MsgIdentifier=251592832  MsgLength=8  SignalInfo={'AngleXAxis_128','0','16','LE','unsigned','Standard','0','0.007813','0','0','512.025';'AngularAccelerationXAxis_128','32','16','LE','unsigned','Standard','0','0.03125','-1000','-1000','1047.9688';'AngularVelocityXAxis_128','16','16','LE','unsigned','Standard','0','0.007813','-250','-250','262.025';'CRC_Xaxis_128','56','8','LE','unsigned','Standard','0','1','0','0','255';'Counter_Xaxis_128','48','8','LE','unsigned','Standard','0','1','0','0','255'}  IDPort=off  TimestampPort=off  ErrorPort=off  RemotePort=off  LengthPort=off  StatusPort=off  ApplyMinMax=off
      settings: LibrarySourceBlock=canlib/CAN Unpack  DataFormat=CANdb specified signals
  Terminator : Terminator
  Angle128X : Outport
  AngleVel128X : Outport  Port=2
  wires:
  CAN Unpack/2 -> Terminator/1
  CAN Unpack/1 -> Angle128X/1
  In1/1 -> CAN Unpack/1
  CAN Unpack/3 -> AngleVel128X/1

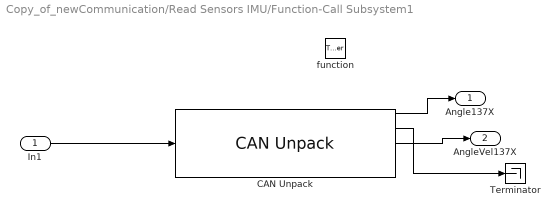
== system Copy_of_newCommunication/Read Sensors IMU/Function-Call Subsystem1 ==
  In1 : Inport
  function : TriggerPort  TriggerType=function-call  VariantControl=(inherit)
  CAN Unpack : canmsglib/CAN Unpack  CANdbFile=C:\Users\Viktor Traktor\Downloads\VolvoExcavator\systemIdentificationVolvo\ec20_kth.dbc  MsgList=IMU_XAxis_137  MsgName=IMU_XAxis_137  MsgIDType=Extended (29-bit identifier)  MsgIdentifier=251592841  MsgLength=8  SignalInfo={'AngleXAxis_137','0','16','LE','unsigned','Standard','0','0.007813','0','0','512.025';'AngularAccelerationXAxis_137','32','16','LE','unsigned','Standard','0','0.03125','-1000','-1000','1047.9688';'AngularVelocityXAxis_137','16','16','LE','unsigned','Standard','0','0.007813','-250','-250','262.025';'CRC_Xaxis_137','56','8','LE','unsigned','Standard','0','1','0','0','255';'Counter_Xaxis_137','48','8','LE','unsigned','Standard','0','1','0','0','255'}  IDPort=off  TimestampPort=off  ErrorPort=off  RemotePort=off  LengthPort=off  StatusPort=off  ApplyMinMax=off
      settings: LibrarySourceBlock=canlib/CAN Unpack  DataFormat=CANdb specified signals
  Terminator : Terminator
  Angle137X : Outport
  AngleVel137X : Outport  Port=2
  wires:
  CAN Unpack/2 -> Terminator/1
  In1/1 -> CAN Unpack/1
  CAN Unpack/1 -> Angle137X/1
  CAN Unpack/3 -> AngleVel137X/1

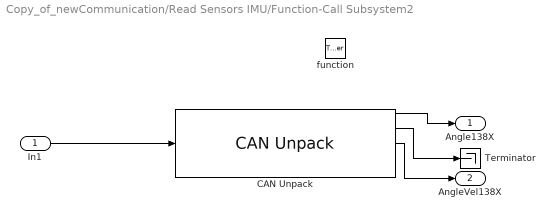
== system Copy_of_newCommunication/Read Sensors IMU/Function-Call Subsystem2 ==
  In1 : Inport
  function : TriggerPort  TriggerType=function-call  VariantControl=(inherit)
  CAN Unpack : canmsglib/CAN Unpack  CANdbFile=C:\Users\Viktor Traktor\Downloads\VolvoExcavator\systemIdentificationVolvo\ec20_kth.dbc  MsgList=IMU_XAxis_138  MsgName=IMU_XAxis_138  MsgIDType=Extended (29-bit identifier)  MsgIdentifier=251592842  MsgLength=8  SignalInfo={'AngleXAxis_138','0','16','LE','unsigned','Standard','0','0.007813','0','0','512.025';'AngularAccelerationXAxis_138','32','16','LE','unsigned','Standard','0','0.03125','-1000','-1000','1047.9688';'AngularVelocityXAxis_138','16','16','LE','unsigned','Standard','0','0.007813','-250','-250','262.025';'CRC_Xaxis_138','56','8','LE','unsigned','Standard','0','1','0','0','255';'Counter_Xaxis_138','48','8','LE','unsigned','Standard','0','1','0','0','255'}  IDPort=off  TimestampPort=off  ErrorPort=off  RemotePort=off  LengthPort=off  StatusPort=off  ApplyMinMax=off
      settings: LibrarySourceBlock=canlib/CAN Unpack  DataFormat=CANdb specified signals
  Terminator : Terminator
  Angle138X : Outport
  AngleVel138X : Outport  Port=2
  wires:
  CAN Unpack/2 -> Terminator/1
  CAN Unpack/1 -> Angle138X/1
  In1/1 -> CAN Unpack/1
  CAN Unpack/3 -> AngleVel138X/1

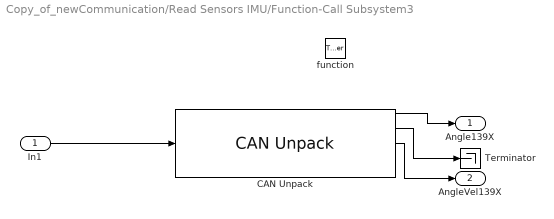
== system Copy_of_newCommunication/Read Sensors IMU/Function-Call Subsystem3 ==
  In1 : Inport
  function : TriggerPort  TriggerType=function-call  VariantControl=(inherit)
  CAN Unpack : canmsglib/CAN Unpack  CANdbFile=C:\Users\Viktor Traktor\Downloads\VolvoExcavator\systemIdentificationVolvo\ec20_kth.dbc  MsgList=IMU_XAxis_139  MsgName=IMU_XAxis_139  MsgIDType=Extended (29-bit identifier)  MsgIdentifier=251592843  MsgLength=8  SignalInfo={'AngleXAxis_139','0','16','LE','unsigned','Standard','0','0.007813','0','0','512.025';'AngularAccelerationXAxis_139','32','16','LE','unsigned','Standard','0','0.03125','-1000','-1000','1047.9688';'AngularVelocityXAxis_139','16','16','LE','unsigned','Standard','0','0.007813','-250','-250','262.025';'CRC_Xaxis_139','56','8','LE','unsigned','Standard','0','1','0','0','255';'Counter_Xaxis_139','48','8','LE','unsigned','Standard','0','1','0','0','255'}  IDPort=off  TimestampPort=off  ErrorPort=off  RemotePort=off  LengthPort=off  StatusPort=off  ApplyMinMax=off
      settings: LibrarySourceBlock=canlib/CAN Unpack  DataFormat=CANdb specified signals
  Terminator : Terminator
  Angle139X : Outport
  AngleVel139X : Outport  Port=2
  wires:
  CAN Unpack/3 -> AngleVel139X/1
  In1/1 -> CAN Unpack/1
  CAN Unpack/1 -> Angle139X/1
  CAN Unpack/2 -> Terminator/1

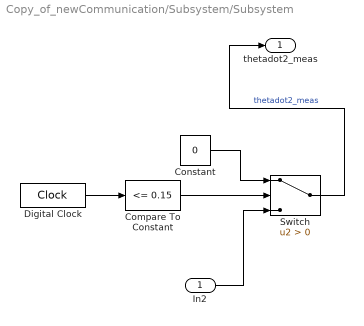
== system Copy_of_newCommunication/Subsystem/Subsystem ==
  In2 : Inport
  Compare To Constant : simulink/Logic and Bit Operations/Compare To Constant  relop=<=  const=0.15  OutDataTypeStr=boolean
  Constant : Constant  Value=0
  Digital Clock : DigitalClock  SampleTime=0.01
  Switch : Switch  Criteria=u2 > Threshold  SaturateOnIntegerOverflow=off  InputSameDT=off
  thetadot2_meas : Outport
  wires:
  In2/1 -> Switch/3
  Digital Clock/1 -> Compare To Constant/1
  Compare To Constant/1 -> Switch/2
  Constant/1 -> Switch/1
  Switch/1 -> thetadot2_meas/1  "thetadot2_meas"

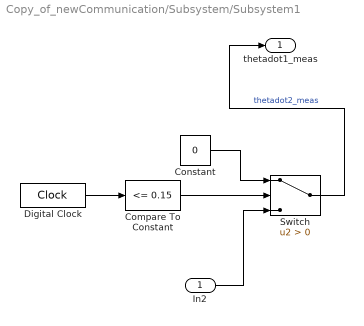
== system Copy_of_newCommunication/Subsystem/Subsystem1 ==
  In2 : Inport
  Compare To Constant : simulink/Logic and Bit Operations/Compare To Constant  relop=<=  const=0.15  OutDataTypeStr=boolean
  Constant : Constant  Value=0
  Digital Clock : DigitalClock  SampleTime=0.01
  Switch : Switch  Criteria=u2 > Threshold  SaturateOnIntegerOverflow=off  InputSameDT=off
  thetadot1_meas : Outport
  wires:
  In2/1 -> Switch/3
  Digital Clock/1 -> Compare To Constant/1
  Compare To Constant/1 -> Switch/2
  Constant/1 -> Switch/1
  Switch/1 -> thetadot1_meas/1  "thetadot2_meas"

== matlab function Copy_of_newCommunication/MATLAB Function1 ==
  data: EncoderPos20X input; angle_20 output; EncoderVel20X input; joint2_pos input; joint2_vel input; velocity_20 output
function [angle_20, velocity_20]= kalman_block(EncoderPos20X, EncoderVel20X, joint2_pos, joint2_vel)
    persistent kf_20
    if isempty(kf_20)
        kf_20 = KalmanFilter(0.01);
    end
    
    kf_20.predict();
    kf_20.update(EncoderPos20X, EncoderVel20X, joint2_pos, joint2_vel);
    
    angle_20 = kf_20.x(1);
    velocity_20 = kf_20.x(2);

end

== matlab function Copy_of_newCommunication/MATLAB Function ==
  data: EncoderPos33X input; angle_33 output; EncoderVel33X input; joint1_pos input; joint1_vel input; velocity_33 output
function [angle_33, velocity_33]= kalman_block(EncoderPos33X, EncoderVel33X, joint1_pos, joint1_vel)
    persistent kf_33
    if isempty(kf_33)
        kf_33 = KalmanFilter(0.01);
    end

    kf_33.predict();
    kf_33.update(EncoderPos33X, EncoderVel33X, joint1_pos, joint1_vel);
    
    angle_33 = kf_33.x(1);
    velocity_33 = kf_33.x(2);

end

== matlab function Copy_of_newCommunication/MATLAB Function2 ==
  data: EncoderPos01X input; angle_01 output; EncoderVel01X input; joint3_pos input; joint3_vel input; velocity_01 output
function [angle_01, velocity_01]= kalman_block(EncoderPos01X, EncoderVel01X, joint3_pos, joint3_vel)
    persistent kf_01
    if isempty(kf_01)
        kf_01 = KalmanFilter(0.01);
    end
    
    kf_01.predict();
    kf_01.update(EncoderPos01X, EncoderVel01X, joint3_pos, joint3_vel);
    
    angle_01 = kf_01.x(1);
    velocity_01 = kf_01.x(2);

end

== matlab function Copy_of_newCommunication/Subsystem/MATLAB Function ==
  data: vx_ref input; thetadot_ref output; vy_ref input; theta1 input; theta2 input
function thetadot_ref = fcn(vx_ref, vy_ref, theta1, theta2)
% Safe version for Simulink — works even when inputs become vectors

vx_ref = vx_ref(1);



if abs(vx_ref)>abs(vy_ref)
    vy_ref = 0;
    flag = 0; %grading mode
else
    vx_ref = 0;
    flag = 1; %lifting mode
end

% Link lengths [m]
L1 = 1903.392e-3;
L2 = 1351.485e-3;

max_joint_vel1 = 0.1;  
max_joint_vel2 = 0.1;

% --- Jacobian ---
J11 = -L1 * sin(theta1) - L2 * sin(theta1 + theta2);
J12 = -L2 * sin(theta1 + theta2);
J21 =  L1 * cos(theta1) + L2 * cos(theta1 + theta2);
J22 =  L2 * cos(theta1 + theta2);

J = [J11 J12; 
     J21 J22];

% --- desired Cartesian velocity vector (2×1) ---
xydot_ref = [vx_ref; vy_ref];


% --- joint velocity reference (IK with pseudoinverse) ---
%thetadot = pinv(J) * xydot_ref;

% --- compute damped least squares inverse (2x2 case) ---
lambda = 0.05;   % damping, tune (0.01..0.2) as needed
JJt = J * J';
inv_term = inv(JJt + lambda^2 * eye(2));
J_dls = J' * inv_term;

thetadot = J_dls * xydot_ref;

% --- clip to joint velocity limits ---
thetadot1 = max(min(thetadot(1), max_joint_vel1), -max_joint_vel1);
thetadot2 = max(min(thetadot(2), max_joint_vel2), -max_joint_vel2);

% --- output vector (2×1) ---
thetadot_ref = [thetadot1; thetadot2];
end

== matlab function Copy_of_newCommunication/MATLAB Function3 ==
  data: x output; x1 output; theta1 input; y output; theta2 input; y1 output; y2 output
function [x,x1,y,y1,y2]= fcn(theta1, theta2)

L1 = 1903.392e-3;
L2 = 1351.485e-3;

x = L1*cos(theta1) + L2*cos(theta1 + theta2);
x1 = L1*cos(theta1) + L2*cos(2*pi - theta1 - theta2);


y = L1*sin(theta1) + L2*sin(theta1 + theta2);
y1 = L1*sin(theta1) - L2*sin(2*pi - theta1 - theta2);
y2 = L1*sin(theta1) + L2*sin(2*pi - theta1 - theta2);

== matlab function Copy_of_newCommunication/MATLAB Function4 ==
  data: theta1dot input; xdot output; theta2dot input; ydot output; theta1 input; theta2 input
function [xdot, ydot] = fcn(theta1dot, theta2dot, theta1, theta2)

% Link lengths [m]
L1 = 1903.392e-3;
L2 = 1351.485e-3;


% --- Jacobian ---
J11 = -L1 * sin(theta1) - L2 * sin(theta1 + theta2);
J12 = -L2 * sin(theta1 + theta2);
J21 =  L1 * cos(theta1) + L2 * cos(theta1 + theta2);
J22 =  L2 * cos(theta1 + theta2);

J = [J11 J12; 
     J21 J22];
xydot = J*[theta1dot; theta2dot];

xdot = xydot(1);
ydot = xydot(2);

== matlab function Copy_of_newCommunication/MATLAB Function5 ==
  data: u input; y output
function y = fcn(u)

y = u;
